simulink model "EHB_speedgoat_R2020a_V1"  (R2020a)
settings: Solver=FixedStepDiscrete  StartTime=0.0  StopTime=inf  FixedStep=0.001  RelTol=1e-3  EnableMultiTasking=on
model workspace (MAT data in the model file):
  A : Simulink.Signal (value not decoded)
  B : Simulink.Signal (value not decoded)
  C : Simulink.Signal (value not decoded)
  D : Simulink.Signal (value not decoded)
  E : Simulink.Signal (value not decoded)
  calin = [-9.96 -7.98 -5.98 -3.99 -1.994 0 1.995 3.992 5.99 7.98 9.97]
  calout = [-10 -8 -6 -4 -2 0 2 4 6 8 10]
symbols that are objects in the model workspace (value not decoded): C, D
undefined symbols (not defined in the file): Com1, none, ts_IO612
libraries: simulink x1436, xpcethercatlib x1223, yisutbxlib_utilities x256, xpcutilitieslib x156, hdlsllib x145, canmsglib x46, speedgoatlib_IO602_4 x11, speedgoatlib_IO611 x7, slrttcplib x4, CanManageLib x3, slrtlib x3, xpcseriallib x2
(part 20 of 30)

== system EHB_speedgoat_R2020a_V1/保留/TIF_06/CB1032_2/DIO/DI ==
  Bit Slice high0 : hdlsllib/Logic and Bit Operations/Bit Slice  lidx=0  ridx=0
      settings: SourceProductBaseCode=SL
  Bit Slice high1 : hdlsllib/Logic and Bit Operations/Bit Slice  lidx=1  ridx=1
      settings: SourceProductBaseCode=SL
  Bit Slice high10 : hdlsllib/Logic and Bit Operations/Bit Slice  lidx=10  ridx=10
      settings: SourceProductBaseCode=SL
  Bit Slice high11 : hdlsllib/Logic and Bit Operations/Bit Slice  lidx=11  ridx=11
      settings: SourceProductBaseCode=SL
  Bit Slice high12 : hdlsllib/Logic and Bit Operations/Bit Slice  lidx=12  ridx=12
      settings: SourceProductBaseCode=SL
  Bit Slice high13 : hdlsllib/Logic and Bit Operations/Bit Slice  lidx=13  ridx=13
      settings: SourceProductBaseCode=SL
  Bit Slice high14 : hdlsllib/Logic and Bit Operations/Bit Slice  lidx=14  ridx=14
      settings: SourceProductBaseCode=SL
  Bit Slice high15 : hdlsllib/Logic and Bit Operations/Bit Slice  lidx=15  ridx=15
      settings: SourceProductBaseCode=SL
  Bit Slice high2 : hdlsllib/Logic and Bit Operations/Bit Slice  lidx=2  ridx=2
      settings: SourceProductBaseCode=SL
  Bit Slice high3 : hdlsllib/Logic and Bit Operations/Bit Slice  lidx=3  ridx=3
      settings: SourceProductBaseCode=SL
  Bit Slice high4 : hdlsllib/Logic and Bit Operations/Bit Slice  lidx=4  ridx=4
      settings: SourceProductBaseCode=SL
  Bit Slice high5 : hdlsllib/Logic and Bit Operations/Bit Slice  lidx=5  ridx=5
      settings: SourceProductBaseCode=SL
  Bit Slice high6 : hdlsllib/Logic and Bit Operations/Bit Slice  lidx=6  ridx=6
      settings: SourceProductBaseCode=SL
  Bit Slice high7 : hdlsllib/Logic and Bit Operations/Bit Slice  lidx=7  ridx=7
      settings: SourceProductBaseCode=SL
  Bit Slice high8 : hdlsllib/Logic and Bit Operations/Bit Slice  lidx=8  ridx=8
      settings: SourceProductBaseCode=SL
  Bit Slice high9 : hdlsllib/Logic and Bit Operations/Bit Slice  lidx=9  ridx=9
      settings: SourceProductBaseCode=SL
  Bit Slice low0 : hdlsllib/Logic and Bit Operations/Bit Slice  lidx=0  ridx=0
      settings: SourceProductBaseCode=SL
  Bit Slice low1 : hdlsllib/Logic and Bit Operations/Bit Slice  lidx=1  ridx=1
      settings: SourceProductBaseCode=SL
  Bit Slice low10 : hdlsllib/Logic and Bit Operations/Bit Slice  lidx=10  ridx=10
      settings: SourceProductBaseCode=SL
  Bit Slice low11 : hdlsllib/Logic and Bit Operations/Bit Slice  lidx=11  ridx=11
      settings: SourceProductBaseCode=SL
  Bit Slice low12 : hdlsllib/Logic and Bit Operations/Bit Slice  lidx=12  ridx=12
      settings: SourceProductBaseCode=SL
  Bit Slice low13 : hdlsllib/Logic and Bit Operations/Bit Slice  lidx=13  ridx=13
      settings: SourceProductBaseCode=SL
  Bit Slice low14 : hdlsllib/Logic and Bit Operations/Bit Slice  lidx=14  ridx=14
      settings: SourceProductBaseCode=SL
  Bit Slice low15 : hdlsllib/Logic and Bit Operations/Bit Slice  lidx=15  ridx=15
      settings: SourceProductBaseCode=SL
  Bit Slice low2 : hdlsllib/Logic and Bit Operations/Bit Slice  lidx=2  ridx=2
      settings: SourceProductBaseCode=SL
  Bit Slice low3 : hdlsllib/Logic and Bit Operations/Bit Slice  lidx=3  ridx=3
      settings: SourceProductBaseCode=SL
  Bit Slice low4 : hdlsllib/Logic and Bit Operations/Bit Slice  lidx=4  ridx=4
      settings: SourceProductBaseCode=SL
  Bit Slice low5 : hdlsllib/Logic and Bit Operations/Bit Slice  lidx=5  ridx=5
      settings: SourceProductBaseCode=SL
  Bit Slice low6 : hdlsllib/Logic and Bit Operations/Bit Slice  lidx=6  ridx=6
      settings: SourceProductBaseCode=SL
  Bit Slice low7 : hdlsllib/Logic and Bit Operations/Bit Slice  lidx=7  ridx=7
      settings: SourceProductBaseCode=SL
  Bit Slice low8 : hdlsllib/Logic and Bit Operations/Bit Slice  lidx=8  ridx=8
      settings: SourceProductBaseCode=SL
  Bit Slice low9 : hdlsllib/Logic and Bit Operations/Bit Slice  lidx=9  ridx=9
      settings: SourceProductBaseCode=SL
  DI_{1..32} (32 alike) : Gain
  DTCB CH_17_32 : DataTypeConversion  OutDataTypeStr=uint16
  DTCB CH_1_16 : DataTypeConversion  OutDataTypeStr=uint16
  EtherCAT PDO Receive1 : xpcethercatlib/EtherCAT PDO Receive  Priority=2  sig_name=Box 2 (YISUWORLD_Dig).PDOGetValue process data mapping.DIL  sig_offset=3080  sig_type=uint16  type_size=16  sig_dim=1  device_id=0  sample_time=0.001000
      settings: SourceProductBaseCode=XP
  EtherCAT PDO Receive2 : xpcethercatlib/EtherCAT PDO Receive  Priority=2  sig_name=Box 2 (YISUWORLD_Dig).PDOGetValue process data mapping.DIH  sig_offset=3064  sig_type=uint16  type_size=16  sig_dim=1  device_id=0  sample_time=0.001000
      settings: SourceProductBaseCode=XP
  DI_CH1 : Outport
  DI_CH2 : Outport  Port=2
  DI_CH3 : Outport  Port=3
  DI_CH4 : Outport  Port=4
  DI_CH5 : Outport  Port=5
  DI_CH6 : Outport  Port=6
  DI_CH7 : Outport  Port=7
  DI_CH8 : Outport  Port=8
  DI_CH9 : Outport  Port=9
  DI_CH10 : Outport  Port=10
  DI_CH11 : Outport  Port=11
  DI_CH12 : Outport  Port=12
  DI_CH13 : Outport  Port=13
  DI_CH14 : Outport  Port=14
  DI_CH15 : Outport  Port=15
  DI_CH16 : Outport  Port=16
  DI_CH17 : Outport  Port=17
  DI_CH18 : Outport  Port=18
  DI_CH19 : Outport  Port=19
  DI_CH20 : Outport  Port=20
  DI_CH21 : Outport  Port=21
  DI_CH22 : Outport  Port=22
  DI_CH23 : Outport  Port=23
  DI_CH24 : Outport  Port=24
  DI_CH25 : Outport  Port=25
  DI_CH26 : Outport  Port=26
  DI_CH27 : Outport  Port=27
  DI_CH28 : Outport  Port=28
  DI_CH29 : Outport  Port=29
  DI_CH30 : Outport  Port=30
  DI_CH31 : Outport  Port=31
  DI_CH32 : Outport  Port=32
  wires:
  EtherCAT PDO Receive1/1 -> DTCB CH_1_16/1
  DTCB CH_1_16/1 -> Bit Slice low0/1, Bit Slice low1/1, Bit Slice low2/1, Bit Slice low3/1, Bit Slice low4/1, Bit Slice low5/1, Bit Slice low6/1, Bit Slice low7/1, Bit Slice low8/1, Bit Slice low9/1, Bit Slice low10/1, Bit Slice low11/1, Bit Slice low12/1, Bit Slice low13/1, Bit Slice low14/1, Bit Slice low15/1
  Bit Slice low0/1 -> DI_1/1
  DI_1/1 -> DI_CH1/1  "DI_CH1"
  Bit Slice low1/1 -> DI_2/1
  DI_2/1 -> DI_CH2/1  "DI_CH2"
  Bit Slice low2/1 -> DI_3/1
  DI_3/1 -> DI_CH3/1  "DI_CH3"
  Bit Slice low3/1 -> DI_4/1
  DI_4/1 -> DI_CH4/1  "DI_CH4"
  Bit Slice low4/1 -> DI_5/1
  DI_5/1 -> DI_CH5/1  "DI_CH5"
  Bit Slice low5/1 -> DI_6/1
  DI_6/1 -> DI_CH6/1  "DI_CH6"
  Bit Slice low6/1 -> DI_7/1
  DI_7/1 -> DI_CH7/1  "DI_CH7"
  Bit Slice low7/1 -> DI_8/1
  DI_8/1 -> DI_CH8/1  "DI_CH8"
  Bit Slice low8/1 -> DI_9/1
  DI_9/1 -> DI_CH9/1  "DI_CH9"
  Bit Slice low9/1 -> DI_10/1
  DI_10/1 -> DI_CH10/1  "DI_CH10"
  Bit Slice low10/1 -> DI_11/1
  DI_11/1 -> DI_CH11/1  "DI_CH11"
  Bit Slice low11/1 -> DI_12/1
  DI_12/1 -> DI_CH12/1  "DI_CH12"
  Bit Slice low12/1 -> DI_13/1
  DI_13/1 -> DI_CH13/1  "DI_CH13"
  Bit Slice low13/1 -> DI_14/1
  DI_14/1 -> DI_CH14/1  "DI_CH14"
  Bit Slice low14/1 -> DI_15/1
  DI_15/1 -> DI_CH15/1  "DI_CH15"
  Bit Slice low15/1 -> DI_16/1
  DI_16/1 -> DI_CH16/1  "DI_CH16"
  EtherCAT PDO Receive2/1 -> DTCB CH_17_32/1
  DTCB CH_17_32/1 -> Bit Slice high0/1, Bit Slice high1/1, Bit Slice high2/1, Bit Slice high3/1, Bit Slice high4/1, Bit Slice high5/1, Bit Slice high6/1, Bit Slice high7/1, Bit Slice high8/1, Bit Slice high9/1, Bit Slice high10/1, Bit Slice high11/1, Bit Slice high12/1, Bit Slice high13/1, Bit Slice high14/1, Bit Slice high15/1
  Bit Slice high0/1 -> DI_17/1
  DI_17/1 -> DI_CH17/1  "DI_CH17"
  Bit Slice high1/1 -> DI_18/1
  DI_18/1 -> DI_CH18/1  "DI_CH18"
  Bit Slice high2/1 -> DI_19/1
  DI_19/1 -> DI_CH19/1  "DI_CH19"
  Bit Slice high3/1 -> DI_20/1
  DI_20/1 -> DI_CH20/1  "DI_CH20"
  Bit Slice high4/1 -> DI_21/1
  DI_21/1 -> DI_CH21/1  "DI_CH21"
  Bit Slice high5/1 -> DI_22/1
  DI_22/1 -> DI_CH22/1  "DI_CH22"
  Bit Slice high6/1 -> DI_23/1
  DI_23/1 -> DI_CH23/1  "DI_CH23"
  Bit Slice high7/1 -> DI_24/1
  DI_24/1 -> DI_CH24/1  "DI_CH24"
  Bit Slice high8/1 -> DI_25/1
  DI_25/1 -> DI_CH25/1  "DI_CH25"
  Bit Slice high9/1 -> DI_26/1
  DI_26/1 -> DI_CH26/1  "DI_CH26"
  Bit Slice high10/1 -> DI_27/1
  DI_27/1 -> DI_CH27/1  "DI_CH27"
  Bit Slice high11/1 -> DI_28/1
  DI_28/1 -> DI_CH28/1  "DI_CH28"
  Bit Slice high12/1 -> DI_29/1
  DI_29/1 -> DI_CH29/1  "DI_CH29"
  Bit Slice high13/1 -> DI_30/1
  DI_30/1 -> DI_CH30/1  "DI_CH30"
  Bit Slice high14/1 -> DI_31/1
  DI_31/1 -> DI_CH31/1  "DI_CH31"
  Bit Slice high15/1 -> DI_32/1
  DI_32/1 -> DI_CH32/1  "DI_CH32"

== system EHB_speedgoat_R2020a_V1/保留/TIF_06/CB1032_2/DIO/DO ==
  DO_CH1 : Inport
  DO_CH2 : Inport  Port=2
  DO_CH3 : Inport  Port=3
  DO_CH4 : Inport  Port=4
  DO_CH5 : Inport  Port=5
  DO_CH6 : Inport  Port=6
  DO_CH7 : Inport  Port=7
  DO_CH8 : Inport  Port=8
  DO_CH9 : Inport  Port=9
  DO_CH10 : Inport  Port=10
  DO_CH11 : Inport  Port=11
  DO_CH12 : Inport  Port=12
  DO_CH13 : Inport  Port=13
  DO_CH14 : Inport  Port=14
  DO_CH15 : Inport  Port=15
  DO_CH16 : Inport  Port=16
  DO_CH17 : Inport  Port=17
  DO_CH18 : Inport  Port=18
  DO_CH19 : Inport  Port=19
  DO_CH20 : Inport  Port=20
  DO_CH21 : Inport  Port=21
  DO_CH22 : Inport  Port=22
  DO_CH23 : Inport  Port=23
  DO_CH24 : Inport  Port=24
  DO_CH25 : Inport  Port=25
  DO_CH26 : Inport  Port=26
  DO_CH27 : Inport  Port=27
  DO_CH28 : Inport  Port=28
  DO_CH29 : Inport  Port=29
  DO_CH30 : Inport  Port=30
  DO_CH31 : Inport  Port=31
  DO_CH32 : Inport  Port=32
  DTCB CH{1..32} (32 alike) : DataTypeConversion  OutDataTypeStr=boolean
  DTCB CH_17_32 : DataTypeConversion
  DTCB CH_1_16 : DataTypeConversion
  EtherCAT PDO Transmit1 : xpcethercatlib/EtherCAT PDO Transmit   Priority=3  sig_name=Box 2 (YISUWORLD_Dig).PDOSet1 process data mapping.DL  sig_offset=2984  sig_type=uint16  type_size=16  sig_dim=1  device_id=0  sample_time=0.001000
      settings: SourceProductBaseCode=XP
  EtherCAT PDO Transmit2 : xpcethercatlib/EtherCAT PDO Transmit   Priority=3  sig_name=Box 2 (YISUWORLD_Dig).PDOSet1 process data mapping.DH  sig_offset=2968  sig_type=uint16  type_size=16  sig_dim=1  device_id=0  sample_time=0.001000
      settings: SourceProductBaseCode=XP
  bit Packing CH_17_32 : xpcutilitieslib/Bit Packing   MaskBitPatterns={[0:0],[1:1],[2:2],[3:3],[4:4],[5:5],[6:6],[7:7],[8:8],[9:9],[10:10],[11:11],[12:12],[13:13],[14:14],[15:15]}  MaskPackDataType=uint16  MaskPackDataSize=[1]
      settings: SourceProductBaseCode=XP
  bit Packing CH_1_16 : xpcutilitieslib/Bit Packing   MaskBitPatterns={[0:0],[1:1],[2:2],[3:3],[4:4],[5:5],[6:6],[7:7],[8:8],[9:9],[10:10],[11:11],[12:12],[13:13],[14:14],[15:15]}  MaskPackDataType=uint16  MaskPackDataSize=[1]
      settings: SourceProductBaseCode=XP
  wires:
  DO_CH1/1 -> DTCB CH1/1
  DO_CH2/1 -> DTCB CH2/1
  DO_CH3/1 -> DTCB CH3/1
  DO_CH4/1 -> DTCB CH4/1
  DO_CH5/1 -> DTCB CH5/1
  DO_CH6/1 -> DTCB CH6/1
  DO_CH7/1 -> DTCB CH7/1
  DO_CH8/1 -> DTCB CH8/1
  DO_CH9/1 -> DTCB CH9/1
  DO_CH10/1 -> DTCB CH10/1
  DO_CH11/1 -> DTCB CH11/1
  DO_CH12/1 -> DTCB CH12/1
  DO_CH13/1 -> DTCB CH13/1
  DO_CH14/1 -> DTCB CH14/1
  DO_CH15/1 -> DTCB CH15/1
  DO_CH16/1 -> DTCB CH16/1
  DTCB CH1/1 -> bit Packing CH_1_16/1
  DTCB CH2/1 -> bit Packing CH_1_16/2
  DTCB CH3/1 -> bit Packing CH_1_16/3
  DTCB CH4/1 -> bit Packing CH_1_16/4
  DTCB CH5/1 -> bit Packing CH_1_16/5
  DTCB CH6/1 -> bit Packing CH_1_16/6
  DTCB CH7/1 -> bit Packing CH_1_16/7
  DTCB CH8/1 -> bit Packing CH_1_16/8
  DTCB CH9/1 -> bit Packing CH_1_16/9
  DTCB CH10/1 -> bit Packing CH_1_16/10
  DTCB CH11/1 -> bit Packing CH_1_16/11
  DTCB CH12/1 -> bit Packing CH_1_16/12
  DTCB CH13/1 -> bit Packing CH_1_16/13
  DTCB CH14/1 -> bit Packing CH_1_16/14
  DTCB CH15/1 -> bit Packing CH_1_16/15
  DTCB CH16/1 -> bit Packing CH_1_16/16
  bit Packing CH_1_16/1 -> DTCB CH_1_16/1
  DTCB CH_1_16/1 -> EtherCAT PDO Transmit1/1
  DO_CH17/1 -> DTCB CH17/1
  DO_CH18/1 -> DTCB CH18/1
  DO_CH19/1 -> DTCB CH19/1
  DO_CH20/1 -> DTCB CH20/1
  DO_CH21/1 -> DTCB CH21/1
  DO_CH22/1 -> DTCB CH22/1
  DO_CH23/1 -> DTCB CH23/1
  DO_CH24/1 -> DTCB CH24/1
  DO_CH25/1 -> DTCB CH25/1
  DO_CH26/1 -> DTCB CH26/1
  DO_CH27/1 -> DTCB CH27/1
  DO_CH28/1 -> DTCB CH28/1
  DO_CH29/1 -> DTCB CH29/1
  DO_CH30/1 -> DTCB CH30/1
  DO_CH31/1 -> DTCB CH31/1
  DO_CH32/1 -> DTCB CH32/1
  DTCB CH17/1 -> bit Packing CH_17_32/1
  DTCB CH18/1 -> bit Packing CH_17_32/2
  DTCB CH19/1 -> bit Packing CH_17_32/3
  DTCB CH20/1 -> bit Packing CH_17_32/4
  DTCB CH21/1 -> bit Packing CH_17_32/5
  DTCB CH22/1 -> bit Packing CH_17_32/6
  DTCB CH23/1 -> bit Packing CH_17_32/7
  DTCB CH24/1 -> bit Packing CH_17_32/8
  DTCB CH25/1 -> bit Packing CH_17_32/9
  DTCB CH26/1 -> bit Packing CH_17_32/10
  DTCB CH27/1 -> bit Packing CH_17_32/11
  DTCB CH28/1 -> bit Packing CH_17_32/12
  DTCB CH29/1 -> bit Packing CH_17_32/13
  DTCB CH30/1 -> bit Packing CH_17_32/14
  DTCB CH31/1 -> bit Packing CH_17_32/15
  DTCB CH32/1 -> bit Packing CH_17_32/16
  bit Packing CH_17_32/1 -> DTCB CH_17_32/1
  DTCB CH_17_32/1 -> EtherCAT PDO Transmit2/1
